simulink model "motion_robot_fal"  (Simulink 10.0)
settings: Solver=FixedStepAuto  StartTime=0.0  StopTime=60  FixedStep=fixedStep  MaxStep=0.2  RelTol=1e-3
undefined symbols (not defined in the file or in its folder): robotDis, sensitivityDis
settings Model: Creator=lixuansong  LastModifiedBy=lixuansong
settings DataIOCC: SaveOutput=off  SignalLogging=off  DSMLogging=off  SaveTime=off
settings OptimizationCC: LifeSpan=auto
settings DebuggingCC: UnderspecifiedInitializationDetection=Simplified  MergeDetectMultiDrivingBlocksExec=error  SFUnexpectedBacktrackingDiag=error  SFNoUnconditionalDefaultTransitionDiag=error  SFExecutionAtInitializationDiag=warning  ArithmeticOperatorsInVariantConditions=error
settings HardwareCC: ProdBitPerPointer=64  ProdBitPerSizeT=64  ProdBitPerPtrDiffT=64  ProdLargestAtomicFloat=Float  ProdIntDivRoundTo=Zero  ProdEndianess=LittleEndian  ProdWordSize=64  ProdHWDeviceType=Intel->x86-64 (Windows64)
settings ModelReferenceCC: PropagateSignalLabelsOutOfModel=on
settings SFSimCC: SimUseLocalCustomCode=on  CustomCodeUndefinedFunction=FilterOut
settings RTWCC: RTWUseLocalCustomCode=on
settings CodeAppCC: StateflowObjectComments=off
settings GRTTargetCC: TargetLangStandard=C99 (ISO)  CombineOutputUpdateFcns=on  GRTInterface=off
settings ConfigComp: CovMetricSettings=dwe  CovHtmlReporting=off  CovSaveCumulativeToWorkspaceVar=off  CovSaveSingleToWorkspaceVar=off

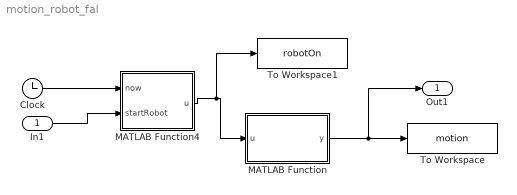
== system motion_robot_fal ==
  In1 : Inport
  Clock : Clock
  MATLAB Function : MATLAB Function  TreatAsAtomicUnit=on
  MATLAB Function4 : MATLAB Function  TreatAsAtomicUnit=on
  To Workspace : ToWorkspace  VariableName=motion  SampleTime=-1
  To Workspace1 : ToWorkspace  VariableName=robotOn  SampleTime=-1
  Out1 : Outport
  wires:
  MATLAB Function4/1(u) -> To Workspace1/1, MATLAB Function/1(u)
  Clock/1 -> MATLAB Function4/1(now)
  MATLAB Function/1(y) -> Out1/1, To Workspace/1
  In1/1 -> MATLAB Function4/2(startRobot)

== matlab function MATLAB Function ==
  data: u input double; y output double; sensitivityDis parameter double; robotDis parameter double
function y = motionDetector(u,sensitivityDis, robotDis)

if robotDis<=sensitivityDis
    y=u;
else
    y=0;
end

== matlab function MATLAB Function4 ==
  data: u output double; now input double; timeRobot parameter double; startRobot input double
function u = controlRobot(now,timeRobot, startRobot)
if now>=startRobot && now<=startRobot+timeRobot
    u=1;
else
    u=0;
end
